simulink model "Model_PI_lambdaD_FOPDT"  (Simulink 9.2)
settings: Solver=FixedStepAuto  StartTime=0.0  StopTime=20  FixedStep=T_s  RelTol=1e-3  EnableMultiTasking=on
values from neighbouring files (symbols this model uses):
  disturb_step_time = handles.disTime    [GUI_Comparison1.m]    (also in GUI_Comparison2.m; GUI_Main.m = str2double(get(handles.edit_disTime,   'string')); function_PI_lambdaD.m = 100; programEx6PILamD.m = 40)
  disturb_step_value = handles.disValue    [GUI_Comparison1.m]    (also in GUI_Comparison2.m; GUI_Main.m = str2double(get(handles.edit_disValue,  'string')); function_PI_lambdaD.m = 0.5; programEx6PILamD.m = 0.5)
  gain = 1    [function_PI_lambdaD.m]
  kdo = Kp*Td    [GUI_Comparison1.m]    (also in GUI_Comparison2.m; GUI_Main.m = handles.kdo; function_PI_lambdaD.m = fpp_kd(j); programEx6PILamD.m = 3.6466)
  kio = Kp/Ti    [GUI_Comparison1.m]    (also in GUI_Comparison2.m; GUI_Main.m = handles.kio; function_PI_lambdaD.m = fpp_ki(j); programEx6PILamD.m = 14.7942)
  kpo = Kp    [GUI_Comparison1.m]    (also in GUI_Comparison2.m; GUI_Main.m = handles.kpo; function_PI_lambdaD.m = fpp_kp(j); programEx6PILamD.m = 0.3835)
  L = handles.L    [GUI_Comparison1.m]    (also in GUI_Comparison2.m; GUI_Main.m; function_PI_lambdaD.m = delay; irid_fod.m = 200)
  ro = fpp_ro(j)    [function_PI_lambdaD.m]
libraries: cstblocks x3
settings Model: Creator=Li Chuang  LastModifiedBy=18764
settings OptimizationCC: InitFltsAndDblsToZero=on
settings DebuggingCC: SaveWithParameterizedLinksMsg=none  SignalResolutionControl=TryResolveAllWithWarning  SolverPrmCheckMsg=warning  MultiTaskDSMMsg=warning  MultiTaskCondExecSysMsg=none  FcnCallInpInsideContextMsg=error  AllowSymbolicDim=off  StateNameClashWarn=none
settings GRTTargetCC: TargetFcnLib=ansi_tfl_tmw.mat  GeneratePreprocessorConditionals=Use local settings

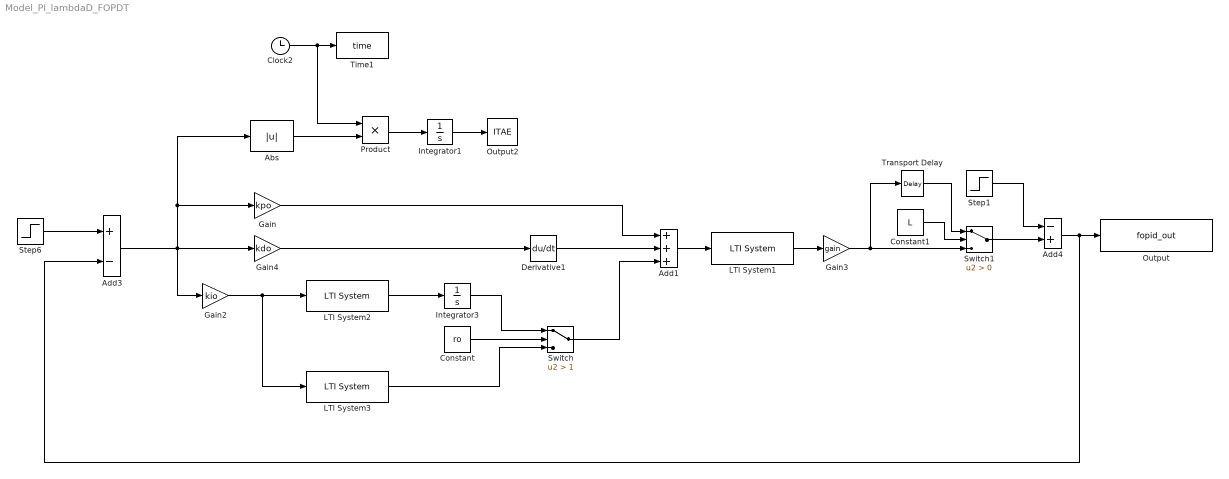
== system Model_PI_lambdaD_FOPDT ==
  Abs : Abs
  Add1 : Sum  Inputs=+++  SaturateOnIntegerOverflow=on  OutDataTypeStr=Inherit: Same as first input
  Add3 : Sum  Inputs=+-  SaturateOnIntegerOverflow=on  OutDataTypeStr=Inherit: Same as first input
  Add4 : Sum  Inputs=-+  SaturateOnIntegerOverflow=on  OutDataTypeStr=Inherit: Same as first input
  Clock2 : Clock
      settings: Decimation=100
  Constant : Constant  Value=ro
  Constant1 : Constant  Value=L
  Derivative1 : Derivative
  Gain : Gain  Gain=kpo
  Gain2 : Gain  Gain=kio
  Gain3 : Gain  Gain=gain
  Gain4 : Gain  Gain=kdo
  Integrator1 : Integrator
  Integrator3 : Integrator
  LTI System1 : cstblocks/LTI System  sys=Gp  IC=[]
  LTI System2 : cstblocks/LTI System  sys=dfod  IC=[]
  LTI System3 : cstblocks/LTI System  sys=dfod  IC=[]
  Output : ToWorkspace  VariableName=fopid_out  SampleTime=-1
  Output2 : ToWorkspace  VariableName=ITAE  SampleTime=-1
  Product : Product
  Step1 : Step  Time=disturb_step_time  After=disturb_step_value
  Step6 : Step  Time=0
  Switch : Switch  Criteria=u2 > Threshold  Threshold=1
  Switch1 : Switch  Criteria=u2 > Threshold
  Time1 : ToWorkspace  VariableName=time  SampleTime=-1
  Transport Delay : TransportDelay  DelayTime=L
  wires:
  Gain/1 -> Add1/1
  LTI System1/1 -> Gain3/1
  Constant1/1 -> Switch1/2
  Transport Delay/1 -> Switch1/1
  Gain3/1 -> Transport Delay/1, Switch1/3
  Gain4/1 -> Derivative1/1
  Derivative1/1 -> Add1/2
  Switch/1 -> Add1/3
  Step6/1 -> Add3/1
  Clock2/1 -> Product/1, Time1/1
  Abs/1 -> Product/2
  Product/1 -> Integrator1/1
  Integrator1/1 -> Output2/1
  Step1/1 -> Add4/1
  Add1/1 -> LTI System1/1
  Switch1/1 -> Add4/2
  Add4/1 -> Add3/2, Output/1
  LTI System3/1 -> Switch/3
  LTI System2/1 -> Integrator3/1
  Gain2/1 -> LTI System3/1, LTI System2/1
  Constant/1 -> Switch/2
  Integrator3/1 -> Switch/1
  Add3/1 -> Gain/1, Abs/1, Gain2/1, Gain4/1
